simulink model "controller_test"  (R2015a)
settings: Solver=ode5  StartTime=0.0  StopTime=1  FixedStep=5e-5  RelTol=1e-3
values from neighbouring files (symbols this model uses):
  Ak = inv(P12)*(A_hat-P12*Bk*Cy*Q11-P11*Bp*Ck*Q12'-P11*(Ap+Bp*Dk*Cy)*Q11)*inv(Q12')    [finding_Q12P12.m]    (also in main_matlab_LMI_Theorem4.m; main_matlab_LMI_Theorem5.m)
  Bk = inv(P12)*(B_hat-P11*Bp*Dk)    [finding_Q12P12.m]    (also in main_matlab_LMI_Theorem4.m; main_matlab_LMI_Theorem5.m)
  Ck = (C_hat-Dk*Cy*Q11)*inv(Q12')    [finding_Q12P12.m]    (also in main_matlab_LMI_Theorem4.m; main_matlab_LMI_Theorem5.m)
  Dk = D_hat    [finding_Q12P12.m]    (also in main_matlab_LMI_Theorem4.m; main_matlab_LMI_Theorem5.m)
undefined symbols (not defined in the file or in its folder): Af, Bf, Cf, Hf
settings Model: Creator=p4wp4w  LastModifiedBy=Ablah

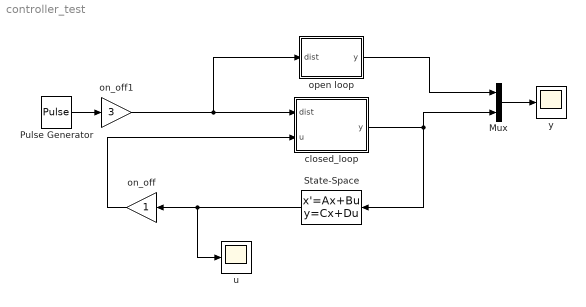
== system controller_test ==
  Mux : Mux  Inputs=2
  Pulse Generator : DiscretePulseGenerator  PulseType=Time based  Period=0.5  PulseWidth=10
  State-Space : StateSpace  A=Ak  B=Bk  C=Ck  D=Dk  X0=0
  closed_loop : Subsystem
  on_off : Gain
  on_off1 : Gain  Gain=3
  open loop : Subsystem
  u : Scope
      settings: YMin=-12.5  YMax=12.5
  y : Scope
      settings: ShowLegends=on  YMin=-3  YMax=3
  wires:
  State-Space/1 -> u/1, on_off/1
  closed_loop/1(y) -> State-Space/1, Mux/2
  Pulse Generator/1 -> on_off1/1
  on_off/1 -> closed_loop/2(u)
  open loop/1(y) -> Mux/1
  Mux/1 -> y/1
  on_off1/1 -> open loop/1(dist), closed_loop/1(dist)

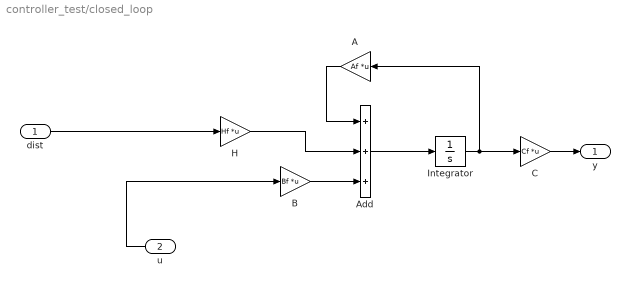
== system controller_test/closed_loop ==
  dist : Inport
  u : Inport  Port=2
  A : Gain  Gain=Af  Multiplication=Matrix(K*u)
  Add : Sum  Inputs=+++
  B : Gain  Gain=Bf  Multiplication=Matrix(K*u)
  C : Gain  Gain=Cf  Multiplication=Matrix(K*u)
  H : Gain  Gain=Hf  Multiplication=Matrix(K*u)
  Integrator : Integrator
  y : Outport
  wires:
  u/1 -> B/1
  dist/1 -> H/1
  H/1 -> Add/2
  C/1 -> y/1
  Integrator/1 -> C/1, A/1
  B/1 -> Add/3
  A/1 -> Add/1
  Add/1 -> Integrator/1

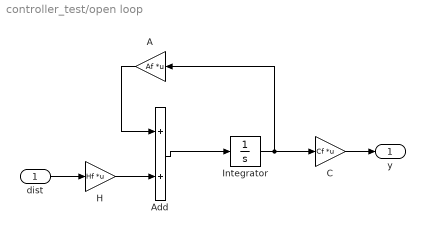
== system controller_test/open loop ==
  dist : Inport
  A : Gain  Gain=Af  Multiplication=Matrix(K*u)
  Add : Sum
  C : Gain  Gain=Cf  Multiplication=Matrix(K*u)
  H : Gain  Gain=Hf  Multiplication=Matrix(K*u)
  Integrator : Integrator
  y : Outport
  wires:
  Add/1 -> Integrator/1
  A/1 -> Add/1
  Integrator/1 -> A/1, C/1
  C/1 -> y/1
  H/1 -> Add/2
  dist/1 -> H/1
